simulink model "servoControllerHydProto"  (R2021b)
settings: Solver=FixedStepDiscrete  StartTime=0.0  StopTime=10.0  FixedStep=1e-3  RelTol=1e-3
undefined symbols (not defined in the file): IO682
libraries: speedgoatlib_IO682 x14, slrealtimeloglib x7, speedgoatlib_IO421 x3, speedgoatlib_IO107 x2, speedgoatlib_IO204 x2, simulink x1
settings Model: Creator=ACH  LastModifiedBy=ACH
settings SolverCC: ConcurrentTasks=on  PositivePriorityOrder=on
settings OptimizationCC: BlockReduction=off  OptimizeBlockIOStorage=off
settings DebuggingCC: TasksWithSamePriorityMsg=none
settings HardwareCC: ProdBitPerLong=64  ProdLongLongMode=on  ProdHWDeviceType=Intel->x86-64 (Linux 64)
settings RTWCC: Description=Simulink Real-Time  SystemTargetFile=slrealtime.tlc  TemplateMakefile=slrealtime_default_tmf  Toolchain=Simulink Real-Time Toolchain  BuildConfiguration=Faster Runs  CodeExecutionProfiling=on  TargetLang=C++

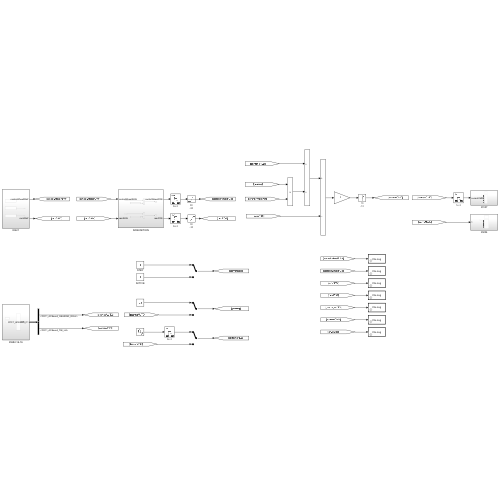
[thumbnail: Simulink's stored preview of the top-level diagram]
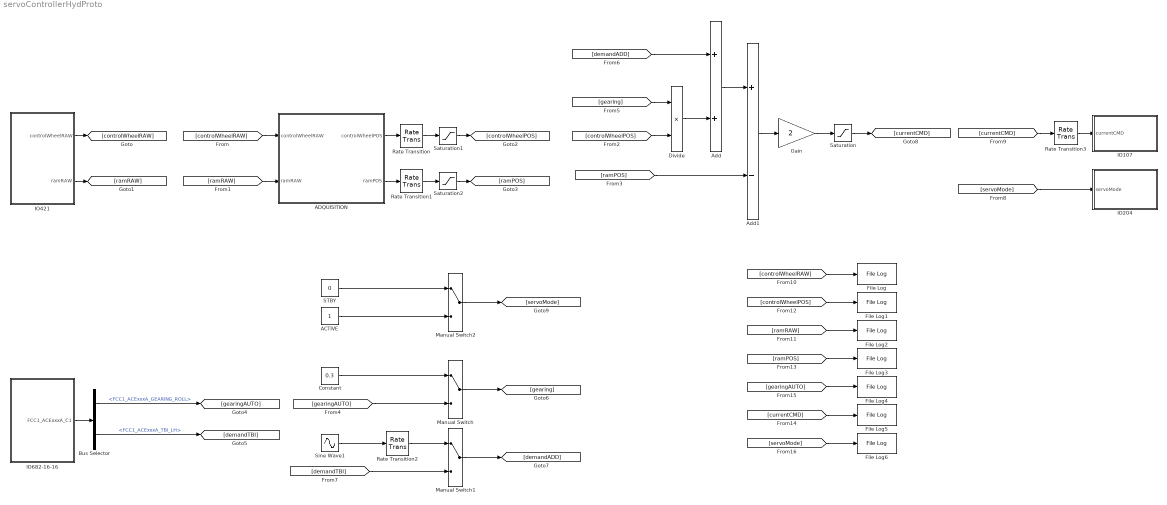
== system servoControllerHydProto ==
  ACTIVE : Constant
  ADQUISITION : Subsystem
  Add : Sum
  Add1 : Sum  Inputs=+-
  Bus Selector : BusSelector  OutputSignals=FCC1_ACExxxA_GEARING_ROLL,FCC1_ACExxxA_TBI_LH
  Constant : Constant  Value=0.3
  Divide : Product  Inputs=**
  File Log{,1..6} (7 alike) : slrealtimeloglib/File Log  decimation=1
      settings: SourceProductBaseCode=XP
  Gain : Gain  Gain=2
  IO107 : Subsystem
  IO204 : Subsystem
  IO421 : Subsystem
  IO682-16-16 : Subsystem
  Manual Switch : ManualSwitch
  Manual Switch1 : ManualSwitch
  Manual Switch2 : ManualSwitch
  Rate Transition : RateTransition  OutPortSampleTime=8e-3
      settings: AttributesFormatString=%<OutPortSampleTime>
  Rate Transition1 : RateTransition  OutPortSampleTime=8e-3
      settings: AttributesFormatString=%<OutPortSampleTime>
  Rate Transition2 : RateTransition  OutPortSampleTime=8e-3
      settings: AttributesFormatString=%<OutPortSampleTime>
  Rate Transition3 : RateTransition  OutPortSampleTime=1e-3
      settings: AttributesFormatString=%<OutPortSampleTime>
  STBY : Constant  Value=0
  Saturation : Saturate  UpperLimit=10  LowerLimit=-10
      settings: AttributesFormatString=|
      | %<UpperLimit>
      | %<LowerLimit>
  Saturation1 : Saturate  UpperLimit=80  LowerLimit=-80
      settings: AttributesFormatString=|
      | %<UpperLimit>
      | %<LowerLimit>
  Saturation2 : Saturate  UpperLimit=30  LowerLimit=-30
      settings: AttributesFormatString=|
      | %<UpperLimit>
      | %<LowerLimit>
  Sine Wave1 : Sin  Amplitude=10  Frequency=2*pi*5  SampleTime=1e-3
  wires:
  IO421/1(controlWheelRAW) -> [controlWheelRAW]
  IO421/2(ramRAW) -> [ramRAW]
  [controlWheelRAW] -> ADQUISITION/1(controlWheelRAW)
  [ramRAW] -> ADQUISITION/2(ramRAW)
  ADQUISITION/1(controlWheelPOS) -> Rate Transition/1
  ADQUISITION/2(ramPOS) -> Rate Transition1/1
  Bus Selector/1 -> [gearingAUTO]  "<FCC1_ACExxxA_GEARING_ROLL>"
  Bus Selector/2 -> [demandTBI]  "<FCC1_ACExxxA_TBI_LH>"
  IO682-16-16/1(FCC1_ACExxxA_C1) -> Bus Selector/1
  [controlWheelPOS] -> Divide/2
  [gearingAUTO] -> Manual Switch/2
  Constant/1 -> Manual Switch/1
  Manual Switch/1 -> [gearing]
  [gearing] -> Divide/1
  Divide/1 -> Add/2
  Manual Switch1/1 -> [demandADD]
  Sine Wave1/1 -> Rate Transition2/1
  [demandTBI] -> Manual Switch1/2
  [demandADD] -> Add/1
  Add/1 -> Add1/1
  [ramPOS] -> Add1/2
  Add1/1 -> Gain/1
  Gain/1 -> Saturation/1
  Saturation/1 -> [currentCMD]
  Rate Transition/1 -> Saturation1/1
  Manual Switch2/1 -> [servoMode]
  STBY/1 -> Manual Switch2/1
  ACTIVE/1 -> Manual Switch2/2
  [currentCMD] -> Rate Transition3/1
  Rate Transition2/1 -> Manual Switch1/1
  Rate Transition3/1 -> IO107/1(currentCMD)
  [servoMode] -> IO204/1(servoMode)
  Saturation1/1 -> [controlWheelPOS]
  Rate Transition1/1 -> Saturation2/1
  Saturation2/1 -> [ramPOS]
  [controlWheelRAW] -> File Log/1
  [controlWheelPOS] -> File Log1/1
  [ramRAW] -> File Log2/1
  [ramPOS] -> File Log3/1
  [gearingAUTO] -> File Log4/1
  [currentCMD] -> File Log5/1
  [servoMode] -> File Log6/1

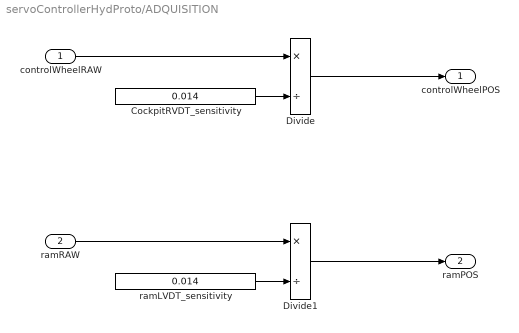
== system servoControllerHydProto/ADQUISITION ==
  controlWheelRAW : Inport
  ramRAW : Inport  Port=2
  CockpitRVDT_sensitivity : Constant  Value=0.014
  Divide : Product  Inputs=*/
  Divide1 : Product  Inputs=*/
  ramLVDT_sensitivity : Constant  Value=0.014
  controlWheelPOS : Outport
  ramPOS : Outport  Port=2
  wires:
  ramRAW/1 -> Divide1/1
  Divide1/1 -> ramPOS/1
  ramLVDT_sensitivity/1 -> Divide1/2
  CockpitRVDT_sensitivity/1 -> Divide/2
  controlWheelRAW/1 -> Divide/1
  Divide/1 -> controlWheelPOS/1

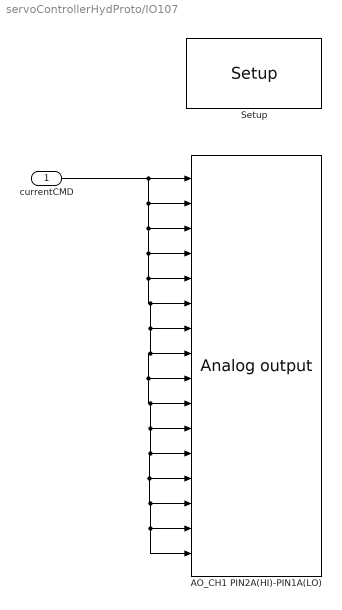
== system servoControllerHydProto/IO107 ==
  currentCMD : Inport
  AO_CH1 PIN2A(HI)-PIN1A(LO) : speedgoatlib_IO107/Analog output  id=1  ts=1e-3  index=[1 2 3 4 5 6 7 8 9 10 11 12 13 14 15 16]  channels=[1 2 3 4 5 6 7 8 9 10 11 12 13 14 15 16]  range=1  pciSlot=-1
      settings: SourceProductName=Simulink Real-Time: Speedgoat Library
  Setup : speedgoatlib_IO107/Setup  group=Module setup  id=1  range=+-10V  triggerSignal=LVDS  groundSense=off  cal=on  pciSlot=-1  daChannel=[1:16]  daInitValue=[0]  daReset=[1]
      settings: SourceProductName=Simulink Real-Time: Speedgoat Library
  wires:
  currentCMD/1 -> AO_CH1 PIN2A(HI)-PIN1A(LO)/6, AO_CH1 PIN2A(HI)-PIN1A(LO)/7, AO_CH1 PIN2A(HI)-PIN1A(LO)/8, AO_CH1 PIN2A(HI)-PIN1A(LO)/9, AO_CH1 PIN2A(HI)-PIN1A(LO)/10, AO_CH1 PIN2A(HI)-PIN1A(LO)/11, AO_CH1 PIN2A(HI)-PIN1A(LO)/12, AO_CH1 PIN2A(HI)-PIN1A(LO)/13, AO_CH1 PIN2A(HI)-PIN1A(LO)/14, AO_CH1 PIN2A(HI)-PIN1A(LO)/16, AO_CH1 PIN2A(HI)-PIN1A(LO)/15, AO_CH1 PIN2A(HI)-PIN1A(LO)/5, AO_CH1 PIN2A(HI)-PIN1A(LO)/4, AO_CH1 PIN2A(HI)-PIN1A(LO)/3, AO_CH1 PIN2A(HI)-PIN1A(LO)/2, AO_CH1 PIN2A(HI)-PIN1A(LO)/1

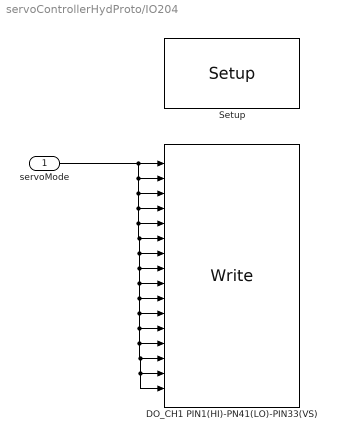
== system servoControllerHydProto/IO204 ==
  servoMode : Inport
  DO_CH1 PIN1(HI)-PN41(LO)-PIN33(VS) : speedgoatlib_IO204/Write  id=1  portType=16 ports of type double  ts=-1  pciSlot=-1
      settings: SourceProductName=Simulink Real-Time: Speedgoat Library
  Setup : speedgoatlib_IO204/Setup  group=Digital output setup  id=1  pciSlot=-1  debounceEnable=on  debounceValue=0.001/10  reset=[0]  value=[0]
      settings: SourceProductName=Simulink Real-Time: Speedgoat Library
  wires:
  servoMode/1 -> DO_CH1 PIN1(HI)-PN41(LO)-PIN33(VS)/16, DO_CH1 PIN1(HI)-PN41(LO)-PIN33(VS)/15, DO_CH1 PIN1(HI)-PN41(LO)-PIN33(VS)/14, DO_CH1 PIN1(HI)-PN41(LO)-PIN33(VS)/13, DO_CH1 PIN1(HI)-PN41(LO)-PIN33(VS)/12, DO_CH1 PIN1(HI)-PN41(LO)-PIN33(VS)/11, DO_CH1 PIN1(HI)-PN41(LO)-PIN33(VS)/10, DO_CH1 PIN1(HI)-PN41(LO)-PIN33(VS)/9, DO_CH1 PIN1(HI)-PN41(LO)-PIN33(VS)/8, DO_CH1 PIN1(HI)-PN41(LO)-PIN33(VS)/7, DO_CH1 PIN1(HI)-PN41(LO)-PIN33(VS)/6, DO_CH1 PIN1(HI)-PN41(LO)-PIN33(VS)/5, DO_CH1 PIN1(HI)-PN41(LO)-PIN33(VS)/4, DO_CH1 PIN1(HI)-PN41(LO)-PIN33(VS)/3, DO_CH1 PIN1(HI)-PN41(LO)-PIN33(VS)/2, DO_CH1 PIN1(HI)-PN41(LO)-PIN33(VS)/1

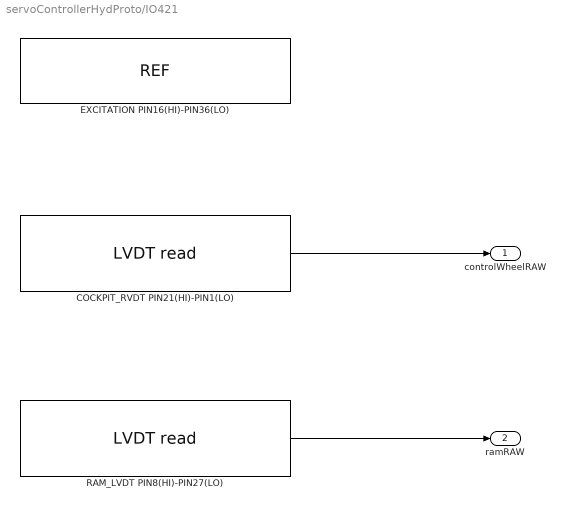
== system servoControllerHydProto/IO421 ==
  COCKPIT_RVDT PIN21(HI)-PIN1(LO) : speedgoatlib_IO421/LVDT//RVDT/LVDT read  id=1  slot=1  channels=[1:1]  wiring=[0]  expectedVLL=[7*0.733/2]  expectedVREF=[7]  ts=1e-3  pciSlot=-1
      settings: SourceProductName=Simulink Real-Time: Speedgoat I/O Blockset
  EXCITATION PIN16(HI)-PIN36(LO) : speedgoatlib_IO421/W/REF  id=1  slot=3  frequency=2e3  voltage=7  pciSlot=-1
      settings: SourceProductName=Simulink Real-Time: Speedgoat I/O Blockset
  RAM_LVDT PIN8(HI)-PIN27(LO) : speedgoatlib_IO421/LVDT//RVDT/LVDT read  id=1  slot=2  channels=[1:1]  wiring=[0]  expectedVLL=[7*0.67/2]  expectedVREF=[7]  ts=1e-3  pciSlot=-1
      settings: SourceProductName=Simulink Real-Time: Speedgoat I/O Blockset
  controlWheelRAW : Outport
  ramRAW : Outport  Port=2
  wires:
  COCKPIT_RVDT PIN21(HI)-PIN1(LO)/1 -> controlWheelRAW/1
  RAM_LVDT PIN8(HI)-PIN27(LO)/1 -> ramRAW/1

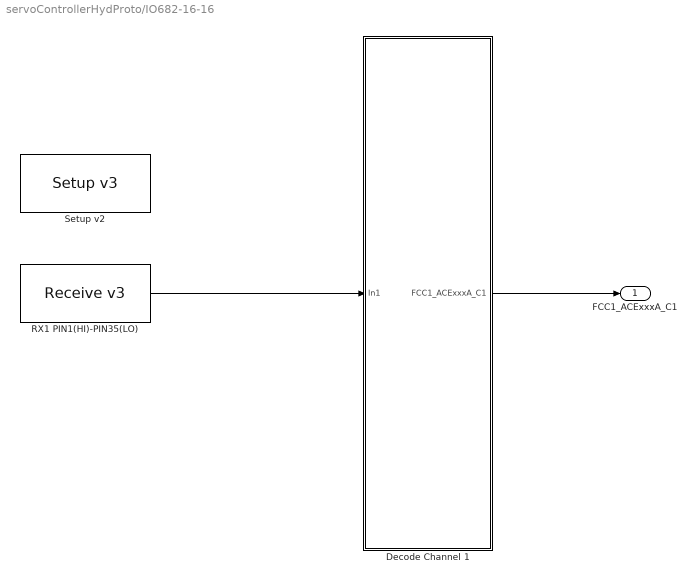
== system servoControllerHydProto/IO682-16-16 ==
  Decode Channel 1 : Subsystem
  RX1 PIN1(HI)-PIN35(LO) : speedgoatlib_IO682/Receive v3   parModuleId=1  parChannel=1  parMaxWords=10  parMinWords=1  parSampleTime=8e-3
      settings: SourceProductName=Speedgoat I/O Blockset
  "Setup v2 " : speedgoatlib_IO682/Setup v3   parModuleId=1  parBoardVariant=IO682-16-16  parPciSlot=-1  parTimerCount=4000*16  parChannelMode=Manual  parInBitRate1=100000  parInBufferMode1=Individual  parInEnable1=on  parInParity1=off  parInInternalWrap1=off  parInBitRate2=100000  parInBufferMode2=Individual  parInEnable2=on  parInParity2=on  parInInternalWrap2=off  parInBitRate3=100000  parInBufferMode3=Individual  parInEnable3=on  parInParity3=on  parInInternalWrap3=off  parInBitRate4=100000  parInBufferMode4=Individual  parInEnable4=on  parInParity4=on  parInInternalWrap4=off  parInBitRate5=100000  parInBufferMode5=Individual  parInEnable5=on  parInParity5=on  parInInternalWrap5=off  parInBitRate6=100000  parInBufferMode6=Individual  parInEnable6=on  parInParity6=on  parInInternalWrap6=off  parInBitRate7=100000  parInBufferMode7=Individual  parInEnable7=on  parInParity7=on  parInInternalWrap7=off  parInBitRate8=100000  parInBufferMode8=Individual  parInEnable8=on  parInParity8=on  parInInternalWrap8=off  parInBitRate9=100000  parInBufferMode9=Individual  parInEnable9=on  parInParity9=on  parInInternalWrap9=off  parInBitRate10=100000  parInBufferMode10=Individual  parInEnable10=on  parInParity10=on  parInInternalWrap10=off  parInBitRate11=100000  parInBufferMode11=Individual  parInEnable11=on  parInParity11=on  parInInternalWrap11=off  parInBitRate12=100000  parInBufferMode12=Individual  parInEnable12=on  parInParity12=on  parInInternalWrap12=off  parInBitRate13=100000  parInBufferMode13=Individual  parInEnable13=on  parInParity13=on  parInInternalWrap13=off  parInBitRate14=100000  parInBufferMode14=Individual  parInEnable14=on  parInParity14=on  parInInternalWrap14=off  parInBitRate15=100000  parInBufferMode15=Individual  parInEnable15=on  parInParity15=on  parInInternalWrap15=off  parInBitRate16=100000  parInBufferMode16=Individual  parInEnable16=on  parInParity16=on  parInInternalWrap16=off  parOutBitRate1=100000  parOutParity1=Odd  parOutProtocolError1=None  parOutEnable1=on  parOutBitRate2=100000  parOutParity2=Odd  parOutProtocolError2=None  parOutEnable2=on  parOutBitRate3=100000  parOutParity3=Odd  parOutProtocolError3=None  parOutEnable3=on  parOutBitRate4=100000  parOutParity4=Odd  parOutProtocolError4=None  parOutEnable4=on  parOutBitRate5=100000  parOutParity5=Odd  parOutProtocolError5=None  parOutEnable5=on  parOutBitRate6=100000  parOutParity6=Odd  parOutProtocolError6=None  parOutEnable6=on  parOutBitRate7=100000  parOutParity7=Odd  parOutProtocolError7=None  parOutEnable7=on  parOutBitRate8=100000  parOutParity8=Odd  parOutProtocolError8=None  parOutEnable8=on  parOutBitRate9=100000  parOutParity9=Odd  parOutProtocolError9=None  parOutEnable9=on  parOutBitRate10=100000  parOutParity10=Odd  parOutProtocolError10=None  parOutEnable10=on  parOutBitRate11=100000  parOutParity11=Odd  parOutProtocolError11=None  parOutEnable11=on  parOutBitRate12=100000  parOutParity12=Odd  parOutProtocolError12=None  parOutEnable12=on  parOutBitRate13=100000  parOutParity13=Odd  parOutProtocolError13=None  parOutEnable13=on  parOutBitRate14=100000  parOutParity14=Odd  parOutProtocolError14=None  parOutEnable14=on  parOutBitRate15=100000  parOutParity15=Odd  parOutProtocolError15=None  parOutEnable15=on  parOutBitRate16=100000  parOutParity16=Odd  parOutProtocolError16=None  parOutEnable16=on  parChConfigFile=''  parScheduleMode=Manual  parScheduledMsgConfigFile=''  parHwDeviceId=hex2dec('0830')  parTimeSource=Internal timer  parChInConfig=[158 8 7 8 1;158 8 7 7 1;158 8 7 7 1;158 8 7 7 1;158 8 7 7 1;158 8 7 7 1;158 8 7 7 1;158 8 7 7 1;158 8 7 7 1;158 8 7 7 1;158 8 7 7 1;158 8 7 7 1;158 8 7 7 1;158 8 7 7 1;158 8 7 7 1;158 8 7 7 1]  parChOutConfig=[158 0 4 7;158 0 4 7;158 0 4 7;158 0 4 7;158 0 4 7;158 0 4 7;158 0 4 7;158 0 4 7;158 0 4 7;158 0 4 7;158 0 4 7;158 0 4 7;158 0 4 7;158 0 4 7;158 0 4 7;158 0 4 7]  parScheduledMessages=0
      settings: SourceProductName=Speedgoat I/O Blockset
  FCC1_ACExxxA_C1 : Outport
  wires:
  RX1 PIN1(HI)-PIN35(LO)/1 -> Decode Channel 1/1(In1)
  Decode Channel 1/1(FCC1_ACExxxA_C1) -> FCC1_ACExxxA_C1/1

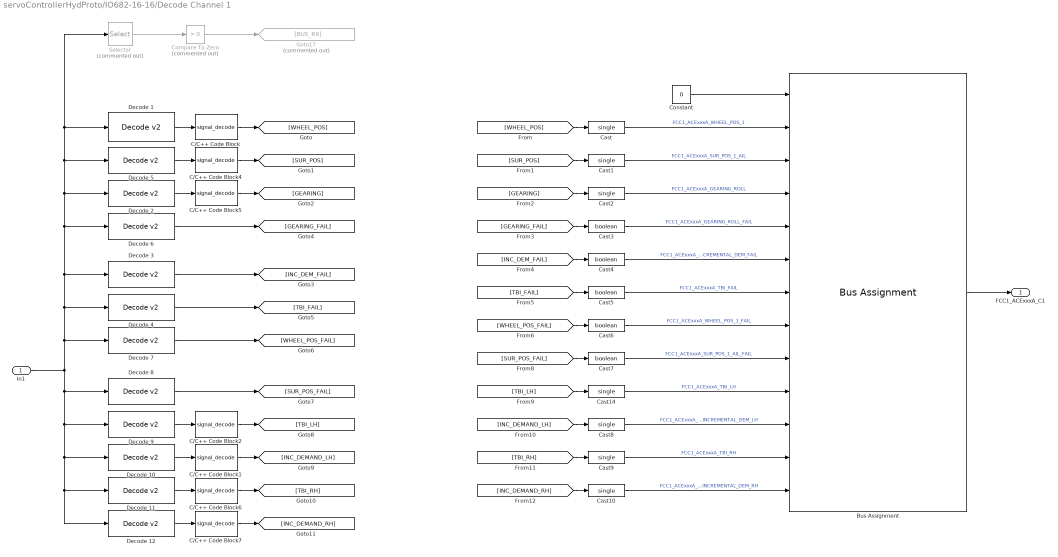
== system servoControllerHydProto/IO682-16-16/Decode Channel 1 ==
  In1 : Inport
  Bus Assignment : BusAssignment  AssignedSignals=FCC1_ACExxxA_WHEEL_POS_1,FCC1_ACExxxA_SUR_POS_1_AIL,FCC1_ACExxxA_GEARING_ROLL,FCC1_ACExxxA_GEARING_ROLL_FAIL,FCC1_ACExxxA_ROLL_INCREMENTAL_DEM_FAIL,FCC1_ACExxxA_TBI_FAIL,FCC1_ACExxxA_WHEEL_POS_1_FAIL,FCC1_ACExxxA_SUR_POS_1_AIL_FAIL,FCC1_ACExxxA_TBI_LH,FCC1_ACExxxA_ROLL_INCREMENTAL_DEM_LH,FCC1_ACExxxA_TBI_RH,FCC1_ACExxxA_ROLL_INCREMENTAL_DEM_RH
  C/C++ Code Block : S-Function  FunctionName=signal_decode  Parameters=6.29922e-1,0,boolean(1),boolean(0),uint32(8)  SFunctionModules=signal_decode_wrapper  SFunctionDeploymentMode=off  EnableBusSupport=off  mask(S-Function Builder){}
      mask help: Simulink:masks:SFunctionBuilder_MD
      mask init:
      | val = [[.9  0.75 0.75 1 1 .9 .9 1]',[1 1 0.75 0.75 .9 .9 1 .9]'];try , sys = get_param(gcb,'SfunBuilderFcnName');if isempty(sys), sys = get_param(gcb,'FunctionName'); end,catch, sys = get_param(gcb,'FunctionName'); end
      settings: CopyFcn=set_param(gcbh,'LinkStatus','none')  OpenFcn=sfunctionwizard(gcbh)
      mask Display:
      | plot(val(:,1),val(:,2))
      | disp(sys)
      | port_label('input',1,'data')
      | port_label('output',1,'out')
  C/C++ Code Block1 : S-Function  FunctionName=signal_decode  Parameters=7.87402E-2,0,boolean(1),boolean(0),uint32(8)  SFunctionModules=signal_decode_wrapper  SFunctionDeploymentMode=off  EnableBusSupport=off  mask(S-Function Builder){}
      mask help: Simulink:masks:SFunctionBuilder_MD
      mask init: same as servoControllerHydProto/IO682-16-16/Decode Channel 1/C/C++ Code Block
      settings: CopyFcn=set_param(gcbh,'LinkStatus','none')  OpenFcn=sfunctionwizard(gcbh)
      mask Display: plot(val(:,1),val(:,2)),disp(sys),port_label('input',1,'data'),port_label('output',1,'out')
  C/C++ Code Block2 : S-Function  FunctionName=signal_decode  Parameters=2.4438E-2,0,boolean(1),boolean(0),uint32(11)  SFunctionModules=signal_decode_wrapper  SFunctionDeploymentMode=off  EnableBusSupport=off  mask(S-Function Builder){}
      mask help: Simulink:masks:SFunctionBuilder_MD
      mask init: same as servoControllerHydProto/IO682-16-16/Decode Channel 1/C/C++ Code Block
      settings: CopyFcn=set_param(gcbh,'LinkStatus','none')  OpenFcn=sfunctionwizard(gcbh)
      mask Display: plot(val(:,1),val(:,2)),disp(sys),port_label('input',1,'data'),port_label('output',1,'out')
  C/C++ Code Block4 : S-Function  FunctionName=signal_decode  Parameters=2.12599E-1,0,boolean(1),boolean(0),uint32(8)  SFunctionModules=signal_decode_wrapper  SFunctionDeploymentMode=off  EnableBusSupport=off  mask(S-Function Builder){}
      mask help: Simulink:masks:SFunctionBuilder_MD
      mask init: same as servoControllerHydProto/IO682-16-16/Decode Channel 1/C/C++ Code Block
      settings: CopyFcn=set_param(gcbh,'LinkStatus','none')  OpenFcn=sfunctionwizard(gcbh)
      mask Display: plot(val(:,1),val(:,2)),disp(sys),port_label('input',1,'data'),port_label('output',1,'out')
  C/C++ Code Block5 : S-Function  FunctionName=signal_decode  Parameters=2.4438E-4,0.2,boolean(0),boolean(0),uint32(10)  SFunctionModules=signal_decode_wrapper  SFunctionDeploymentMode=off  EnableBusSupport=off  mask(S-Function Builder){}
      mask help: Simulink:masks:SFunctionBuilder_MD
      mask init: same as servoControllerHydProto/IO682-16-16/Decode Channel 1/C/C++ Code Block
      settings: CopyFcn=set_param(gcbh,'LinkStatus','none')  OpenFcn=sfunctionwizard(gcbh)
      mask Display: plot(val(:,1),val(:,2)),disp(sys),port_label('input',1,'data'),port_label('output',1,'out')
  C/C++ Code Block6 : S-Function  FunctionName=signal_decode  Parameters=2.4438E-2,0,boolean(1),boolean(0),uint32(11)  SFunctionModules=signal_decode_wrapper  SFunctionDeploymentMode=off  EnableBusSupport=off  mask(S-Function Builder){}
      mask help: Simulink:masks:SFunctionBuilder_MD
      mask init: same as servoControllerHydProto/IO682-16-16/Decode Channel 1/C/C++ Code Block
      settings: CopyFcn=set_param(gcbh,'LinkStatus','none')  OpenFcn=sfunctionwizard(gcbh)
      mask Display: plot(val(:,1),val(:,2)),disp(sys),port_label('input',1,'data'),port_label('output',1,'out')
  C/C++ Code Block7 : S-Function  FunctionName=signal_decode  Parameters=7.87402E-2,0,boolean(1),boolean(0),uint32(8)  SFunctionModules=signal_decode_wrapper  SFunctionDeploymentMode=off  EnableBusSupport=off  mask(S-Function Builder){}
      mask help: Simulink:masks:SFunctionBuilder_MD
      mask init: same as servoControllerHydProto/IO682-16-16/Decode Channel 1/C/C++ Code Block
      settings: CopyFcn=set_param(gcbh,'LinkStatus','none')  OpenFcn=sfunctionwizard(gcbh)
      mask Display: plot(val(:,1),val(:,2)),disp(sys),port_label('input',1,'data'),port_label('output',1,'out')
  Cast{,1..2,8..10,14} (7 alike) : DataTypeConversion  OutDataTypeStr=single
  Cast{3..7} (5 alike) : DataTypeConversion  OutDataTypeStr=boolean
  Compare To Zero : simulink/Logic and Bit Operations/Compare To Zero  Commented=on  relop=>  OutDataTypeStr=boolean
  Constant : Constant  Value=0  OutDataTypeStr=Bus: FCC1_ACExxxA_C1_A  SampleTime=0.008
  Decode 1 : speedgoatlib_IO682/Decode v2   parMode=Custom Data Type  parLabel=55  parDataType=[2]  parResolution=[4096]  parSyncMask=hex2dec('0x0')  parSyncValue=hex2dec('0x0')  parCustomDataType=Raw  parDataLSB=11  parDataMSB=18  parBitPosition=[9, 31]  parScaleBNR=1  parExponent=8  parMantissa=14  parTimeTags=off  parHoldLastVal=on  parStatus=off
      settings: SourceProductName=Simulink Real-Time: Speedgoat I/O Blockset
  Decode 10 : speedgoatlib_IO682/Decode v2   parMode=Custom Data Type  parLabel=163  parDataType=[1]  parResolution=[65536]  parSyncMask=hex2dec('0x0')  parSyncValue=hex2dec('0x0')  parCustomDataType=Raw  parDataLSB=22  parDataMSB=29  parBitPosition=[26]  parScaleBNR=1  parExponent=8  parMantissa=14  parTimeTags=off  parHoldLastVal=on  parStatus=off
      settings: SourceProductName=Simulink Real-Time: Speedgoat I/O Blockset
  Decode 11 : speedgoatlib_IO682/Decode v2   parMode=Custom Data Type  parLabel=231  parDataType=[1]  parResolution=[65536]  parSyncMask=hex2dec('0x0')  parSyncValue=hex2dec('0x0')  parCustomDataType=Raw  parDataLSB=11  parDataMSB=21  parBitPosition=[11]  parScaleBNR=1  parExponent=8  parMantissa=14  parTimeTags=off  parHoldLastVal=on  parStatus=off
      settings: SourceProductName=Simulink Real-Time: Speedgoat I/O Blockset
  Decode 12 : speedgoatlib_IO682/Decode v2   parMode=Custom Data Type  parLabel=231  parDataType=[1]  parResolution=[65536]  parSyncMask=hex2dec('0x0')  parSyncValue=hex2dec('0x0')  parCustomDataType=Raw  parDataLSB=22  parDataMSB=29  parBitPosition=[26]  parScaleBNR=1  parExponent=8  parMantissa=14  parTimeTags=off  parHoldLastVal=on  parStatus=off
      settings: SourceProductName=Simulink Real-Time: Speedgoat I/O Blockset
  Decode 2 : speedgoatlib_IO682/Decode v2   parMode=Custom Data Type  parLabel=112  parDataType=[3]  parResolution=[.1]  parSyncMask=hex2dec('0x0')  parSyncValue=hex2dec('0x0')  parCustomDataType=Raw  parDataLSB=11  parDataMSB=20  parBitPosition=[23]  parScaleBNR=1  parExponent=8  parMantissa=14  parTimeTags=off  parHoldLastVal=on  parStatus=off
      settings: SourceProductName=Simulink Real-Time: Speedgoat I/O Blockset
  Decode 3 : speedgoatlib_IO682/Decode v2   parMode=Custom Data Type  parLabel=112  parDataType=[1]  parResolution=[65536]  parSyncMask=hex2dec('0x0')  parSyncValue=hex2dec('0x0')  parCustomDataType=Discrete  parDataLSB=9  parDataMSB=31  parBitPosition=[24]  parScaleBNR=1  parExponent=8  parMantissa=14  parTimeTags=off  parHoldLastVal=on  parStatus=off
      settings: SourceProductName=Simulink Real-Time: Speedgoat I/O Blockset
  Decode 4 : speedgoatlib_IO682/Decode v2   parMode=Custom Data Type  parLabel=112  parDataType=[1]  parResolution=[1024]  parSyncMask=hex2dec('0x0')  parSyncValue=hex2dec('0x0')  parCustomDataType=Discrete  parDataLSB=12  parDataMSB=25  parBitPosition=[26]  parScaleBNR=1  parExponent=8  parMantissa=14  parTimeTags=off  parHoldLastVal=on  parStatus=off
      settings: SourceProductName=Simulink Real-Time: Speedgoat I/O Blockset
  Decode 5 : speedgoatlib_IO682/Decode v2   parMode=Custom Data Type  parLabel=55  parDataType=[3]  parResolution=[.1]  parSyncMask=hex2dec('0x0')  parSyncValue=hex2dec('0x0')  parCustomDataType=Raw  parDataLSB=19  parDataMSB=26  parBitPosition=[23]  parScaleBNR=1  parExponent=8  parMantissa=14  parTimeTags=off  parHoldLastVal=on  parStatus=off
      settings: SourceProductName=Simulink Real-Time: Speedgoat I/O Blockset
  Decode 6 : speedgoatlib_IO682/Decode v2   parMode=Custom Data Type  parLabel=112  parDataType=[3]  parResolution=[.1]  parSyncMask=hex2dec('0x0')  parSyncValue=hex2dec('0x0')  parCustomDataType=Discrete  parDataLSB=24  parDataMSB=27  parBitPosition=[23]  parScaleBNR=1  parExponent=8  parMantissa=14  parTimeTags=off  parHoldLastVal=on  parStatus=off
      settings: SourceProductName=Simulink Real-Time: Speedgoat I/O Blockset
  Decode 7 : speedgoatlib_IO682/Decode v2   parMode=Custom Data Type  parLabel=112  parDataType=[1]  parResolution=[1024]  parSyncMask=hex2dec('0x0')  parSyncValue=hex2dec('0x0')  parCustomDataType=Discrete  parDataLSB=26  parDataMSB=29  parBitPosition=[28]  parScaleBNR=1  parExponent=8  parMantissa=14  parTimeTags=off  parHoldLastVal=on  parStatus=off
      settings: SourceProductName=Simulink Real-Time: Speedgoat I/O Blockset
  Decode 8 : speedgoatlib_IO682/Decode v2   parMode=Custom Data Type  parLabel=112  parDataType=[1]  parResolution=[65536]  parSyncMask=hex2dec('0x0')  parSyncValue=hex2dec('0x0')  parCustomDataType=Discrete  parDataLSB=9  parDataMSB=31  parBitPosition=[29]  parScaleBNR=1  parExponent=8  parMantissa=14  parTimeTags=off  parHoldLastVal=on  parStatus=off
      settings: SourceProductName=Simulink Real-Time: Speedgoat I/O Blockset
  Decode 9 : speedgoatlib_IO682/Decode v2   parMode=Custom Data Type  parLabel=163  parDataType=[1]  parResolution=[65536]  parSyncMask=hex2dec('0x0')  parSyncValue=hex2dec('0x0')  parCustomDataType=Raw  parDataLSB=11  parDataMSB=21  parBitPosition=[11]  parScaleBNR=1  parExponent=8  parMantissa=14  parTimeTags=off  parHoldLastVal=on  parStatus=off
      settings: SourceProductName=Simulink Real-Time: Speedgoat I/O Blockset
  Goto17 : Goto  Commented=on  GotoTag=BUS_RX
  Selector : Selector  Commented=on  InputPortWidth=11  IndexOptions=Index vector (dialog)  Indices=[1]  OutputSizes=1
  FCC1_ACExxxA_C1 : Outport
  wires:
  Decode 5/1 -> C/C++ Code Block4/1
  Decode 3/1 -> [INC_DEM_FAIL]
  Decode 2/1 -> C/C++ Code Block5/1
  Decode 6/1 -> [GEARING_FAIL]
  Decode 7/1 -> [WHEEL_POS_FAIL]
  Decode 8/1 -> [SUR_POS_FAIL]
  In1/1 -> Decode 6/1, Decode 2/1, Decode 5/1, Selector/1, Decode 1/1, Decode 3/1, Decode 4/1, Decode 7/1, Decode 12/1, Decode 11/1, Decode 10/1, Decode 9/1, Decode 8/1
  Decode 9/1 -> C/C++ Code Block2/1
  Decode 10/1 -> C/C++ Code Block1/1
  Decode 11/1 -> C/C++ Code Block6/1
  Decode 12/1 -> C/C++ Code Block7/1
  [WHEEL_POS] -> Cast/1
  [SUR_POS] -> Cast1/1
  [GEARING] -> Cast2/1
  [INC_DEM_FAIL] -> Cast4/1
  [TBI_FAIL] -> Cast5/1
  [WHEEL_POS_FAIL] -> Cast6/1
  [SUR_POS_FAIL] -> Cast7/1
  [TBI_LH] -> Cast14/1
  [INC_DEMAND_LH] -> Cast8/1
  [TBI_RH] -> Cast9/1
  [INC_DEMAND_RH] -> Cast10/1
  Cast/1 -> Bus Assignment/2  "FCC1_ACExxxA_WHEEL_POS_1"
  Cast1/1 -> Bus Assignment/3  "FCC1_ACExxxA_SUR_POS_1_AIL"
  Cast2/1 -> Bus Assignment/4  "FCC1_ACExxxA_GEARING_ROLL"
  Cast3/1 -> Bus Assignment/5  "FCC1_ACExxxA_GEARING_ROLL_FAIL"
  Cast4/1 -> Bus Assignment/6  "FCC1_ACExxxA_ROLL_INCREMENTAL_DEM_FAIL"
  Cast5/1 -> Bus Assignment/7  "FCC1_ACExxxA_TBI_FAIL"
  Cast6/1 -> Bus Assignment/8  "FCC1_ACExxxA_WHEEL_POS_1_FAIL"
  Cast7/1 -> Bus Assignment/9  "FCC1_ACExxxA_SUR_POS_1_AIL_FAIL"
  Cast8/1 -> Bus Assignment/11  "FCC1_ACExxxA_ROLL_INCREMENTAL_DEM_LH"
  Cast9/1 -> Bus Assignment/12  "FCC1_ACExxxA_TBI_RH"
  Cast10/1 -> Bus Assignment/13  "FCC1_ACExxxA_ROLL_INCREMENTAL_DEM_RH"
  Cast14/1 -> Bus Assignment/10  "FCC1_ACExxxA_TBI_LH"
  Decode 1/1 -> C/C++ Code Block/1
  C/C++ Code Block/1 -> [WHEEL_POS]
  Decode 4/1 -> [TBI_FAIL]
  C/C++ Code Block2/1 -> [TBI_LH]
  Selector/1 -> Compare To Zero/1
  Compare To Zero/1 -> Goto17/1
  C/C++ Code Block4/1 -> [SUR_POS]
  C/C++ Code Block5/1 -> [GEARING]
  C/C++ Code Block1/1 -> [INC_DEMAND_LH]
  C/C++ Code Block6/1 -> [TBI_RH]
  C/C++ Code Block7/1 -> [INC_DEMAND_RH]
  [GEARING_FAIL] -> Cast3/1
  Bus Assignment/1 -> FCC1_ACExxxA_C1/1
  Constant/1 -> Bus Assignment/1
